simulink model "tmp_model_5"  (R2018b)
settings: Solver=VariableStepAuto  StartTime=0.0  StopTime=100  FixedStep=0.001  RelTol=1e-3
libraries: fl_lib x57, sdl_lib x18, nesl_utility x9
(part 1 of 3)
settings Model: Creator=Tanya  LastModifiedBy=Tanya
settings SolverCC: ZeroCrossAlgorithm=Adaptive
settings DebuggingCC: AlgebraicLoopMsg=none  MaskedZcDiagnostic=none  IgnoredZcDiagnostic=none

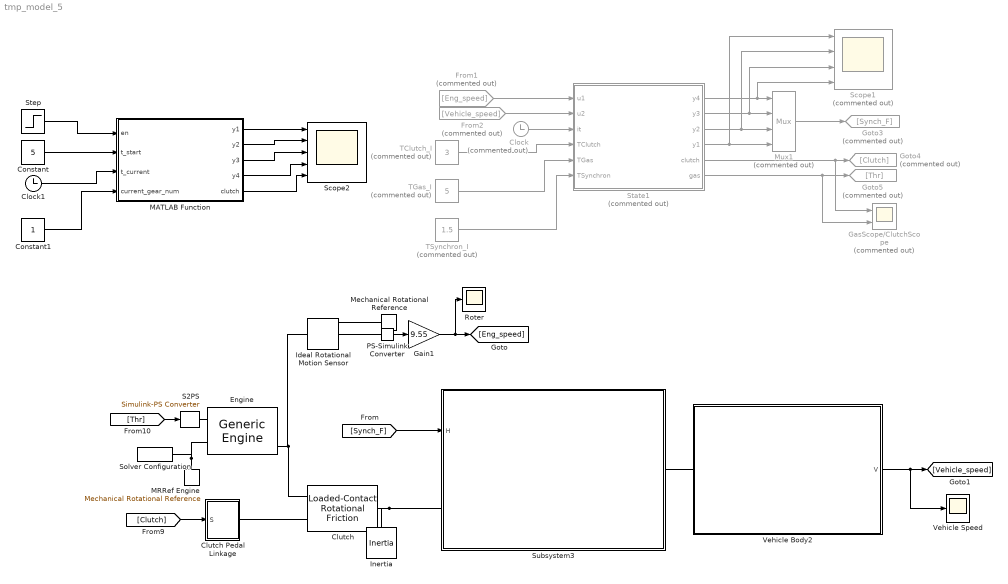
== system tmp_model_5 ==
  Clock : Clock  Commented=on
  Clock1 : Clock
  Clutch : sdl_lib/Brakes & Detents/Rotational/Loaded-Contact Rotational Friction  geometry_model=1  r_eff=300 mm  d_o=150 mm  d_i=100 mm  friction_model=1  mu_coulomb=0.46  mu_w_vector=[ 0 0.1 0.2 0.3 0.4 0.5 1 2 5 10 100 1000 ] rad/s  mu_coulomb_vector=[ 0.29 0.28 0.26 0.22 0.21 0.2 0.2 0.19 0.19 0.19 0.19 0.19 ]  mu_interp_method=1  mu_extrap_method=1  mu_static=0.5  w_tol=0.001 rad/s  force_min=10 N  mu_visc=0 N*m/(rad/s)  initial_state_locked=0  temperature_TLU=[280.0, 300.0, 320.0] K  mu_coulomb_temp_vector=[0.3, 0.28, 0.25]  mu_coulomb_matrix=[0.34, 0.32, 0.3; 0.3, 0.28, 0.25; 0.25, 0.2, 0.15]  mu_static_vector=[0.4, 0.38, 0.36]  thermal_mass=50 kJ/K  T_init=300 K
      settings: SourceProductName=Simscape Driveline  SourceProductBaseCode=LD
  Clutch Pedal Linkage : Subsystem  Tag=PublishSubsystem
      mask Display:
      | color('white')
      | plot(-40,-80);
      | plot(40,40);
      | color('black'),
      | patch([-45 -30 -20 -20 -45],[-90 -90 -75 -55 -90]+20)
      | patch([-30 -10  5 10 20 [20 10 6 -10 -30]-2],[-55 -50 20 25 35 fliplr([-55 -50 20 25 35])-5]);
  Constant : Constant  Value=5
  Constant1 : Constant
  Engine : sdl_lib/Engines/Generic Engine  model_parameterization=1  engine_type=1  P_max=100e3 W  w_P_max=6500 rpm  w_max=8500 rpm  w_min=200 rpm  w_tab=[ 500 1000 2e+3 3e+3 4e+3 5e+3 6e+3 7e+3 ] rpm  trq_tab=[ 380 380 380 380 350 280 200 80 ] N*m  pwr_tab=[ 2e+4 4e+4 7.8e+4 1.2e+5 1.45e+5 1.48e+5 1.25e+5 6e+4 ] W  interp_method=simscape.enum.interpolation.linear  model_inertia=1  inertia=0.16 kg*m^2  initial_velocity=800 rpm  model_time_constant=1  time_constant=0.2 s  T0=0  w_thr=20 rpm  idle_speed=1  idle_speed_reference=800 rpm  tau_controller=.6 s  idle_w_thr=1 rpm  redline=0  redline_speed=5000 rpm  tau_redline=1 s  redline_w_thr=1 rpm  fc_model=0  fc_per_rev=25 mg/rev  displaced_volume=400 cm^3  rev_per_cycle=2  fc_w_tab=[ 1000 2e+3 3e+3 4e+3 5e+3 6e+3 ] rpm  fc_trq_tab=[ 0 80 160 200 240 320 360 400 ] N*m  fc_tab=[ 0.5 0.9 1.4 1.6 1.9 2.7 3.4 4.4; 1 1.7 2.7 3.1 3.6 5 6 7.4; 1.4 2.7 4 4.8 5.6 7.5 8.5 10.5; 2 3.6 5.8 6.7 8 10.4 11.7 13.3; 2.5 4.8 7.9 9.4 10.8 14 16.2 18.6; 3.1 6 10.3 11.9 13.8 18.4 22 26.5 ] g/s  bmep_tab=[ 0 250 500 625 750 1000 1.15e+3 1.25e+3 ] kPa  bsfc_tab=[ 410 380 300 280 270 290 320 380; 410 370 290 270 260 270 285 320; 415 380 290 275 265 270 270 300; 420 390 310 290 285 280 280 285; 430 410 340 320 310 300 310 320; 450 430 370 340 330 330 350 380 ] g/hr/kW  fc_interp_method=simscape.enum.interpolation.linear
      settings: SourceProductName=Simscape Driveline  SourceProductBaseCode=LD
  From1 : From  Commented=on  GotoTag=Eng_speed
  From2 : From  Commented=on  GotoTag=Vehicle_speed
  Gain1 : Gain  Gain=9.55
  GasScope/ClutchScope : Scope  Commented=on  NumInputPorts=2
  Goto3 : Goto  Commented=on  GotoTag=Synch_F
  Goto4 : Goto  Commented=on  GotoTag=Clutch
  Goto5 : Goto  Commented=on  GotoTag=Thr
  Ideal Rotational Motion Sensor : fl_lib/Mechanical/Mechanical Sensors/Ideal Rotational Motion Sensor  offset=0 rad
  Inertia : fl_lib/Mechanical/Rotational Elements/Inertia  inertia=0.005 kg*m^2  w_specify=off  w_priority=High  w=0 rad/s  w_nominal_specify=off  w_nominal_unit=rad/s  w_nominal_value=1  t_specify=off  t_priority=High  t=0 N*m  t_nominal_specify=off  t_nominal_unit=N*m  t_nominal_value=1
  MATLAB Function : MATLAB Function  TreatAsAtomicUnit=on
  MRRef Engine : fl_lib/Mechanical/Rotational Elements/Mechanical Rotational Reference
  Mechanical Rotational Reference : fl_lib/Mechanical/Rotational Elements/Mechanical Rotational Reference
  Mux1 : Mux  Commented=on
  PS-Simulink Converter : nesl_utility/PS-Simulink Converter  PhysicalDomain=network_engine_domain  SubClassName=ps_output  LeftPortType=input  RightPortType=output  PseudoPeriodic=off  Frequencies=[]  Unit=rad/s  AffineConversion=off
  Roter : Scope
  S2PS : nesl_utility/Simulink-PS Converter  PhysicalDomain=network_engine_domain  SubClassName=ps_input  LeftPortType=input  RightPortType=output  PseudoPeriodic=off  Frequencies=[]  NoiseDistribution=none  NoiseParameters=[]  Unit=1  AffineConversion=off  FilteringAndDerivatives=zero  SimscapeFilterOrder=1  InputFilterTimeConstant=.001  UdotUserProvided=0
  Scope1 : Scope  Commented=on  NumInputPorts=4
  Scope2 : Scope  NumInputPorts=5
  Solver Configuration : nesl_utility/Solver Configuration  PhysicalDomain=network_engine_domain  SubClassName=solver  LeftPortType=input  RightPortType=generic  Tones=[]  Harmonics=[]  SimulateNoise=off  Profile=off  UseLocalSampling=off  EnableSwitchedLinearOptims=on  FrequencyDomain=off  UseCCode=off  RelTol=0.001  AbsTol=1e-06  MinStep=1e-09  ToWorkspace=off  RevertToSquareIcSolve=off  NumHomotopyIterations=100  PhasorMode=off  PhasorModeNumHarmonics=1  DoDC=off  ResidualTolerance=1e-9  UseLocalSolver=off  LocalSolverChoice=NE_BACKWARD_EULER_ADVANCER  LocalSolverSampleTime=.001  DoFixedCost=off  MaxNonlinIter=3  MaxModeIter=2  LinearAlgebra=auto  EquationFormulation=NE_TIME_EF  DelaysMemoryBudget=1024  AutomaticFiltering=on  FilteringTimeConstant=0.001  PartitionStorageMethod=AS_NEEDED  PartitionMemoryBudget=1024
  State1 : MATLAB Function  Commented=on  TreatAsAtomicUnit=on
  Step : Step  Time=5  SampleTime=0
  Subsystem3 : Subsystem
      mask Display: image('content_ponizhennaya_peredacha_nizhnyaya_stupen_delitelya2.png');
  TClutch_I : Constant  Commented=on  Value=3
  TGas_I : Constant  Commented=on  Value=5
  TSynchron_I : Constant  Commented=on  Value=1.5
  Vehicle Speed : Scope
  Vehicle Body2 : Subsystem  Tag=PublishSubsystem
      mask Display: image('gazel_avto.png');
  wires:
  [Thr] -> S2PS/1
  [Synch_F] -> Subsystem3/1(H)
  [Clutch] -> Clutch Pedal Linkage/1(S)
  PS-Simulink Converter/1 -> Gain1/1
  Clock/1 -> State1/3(it)
  Mux1/1 -> Goto3/1
  TClutch_I/1 -> State1/4(TClutch)
  TGas_I/1 -> State1/5(TGas)
  TSynchron_I/1 -> State1/6(TSynchron)
  Gain1/1 -> [Eng_speed], Roter/1
  State1/1(y4) -> Scope1/4, Mux1/1
  State1/2(y3) -> Scope1/3, Mux1/2
  State1/3(y2) -> Scope1/2, Mux1/3
  State1/4(y1) -> Scope1/1, Mux1/4
  State1/5(clutch) -> GasScope/ClutchScope/1, Goto4/1
  State1/6(gas) -> GasScope/ClutchScope/2, Goto5/1
  Vehicle Body2/1(V) -> [Vehicle_speed], Vehicle Speed/1
  From1/1 -> State1/1(u1)
  From2/1 -> State1/2(u2)
  Step/1 -> MATLAB Function/1(en)
  Constant/1 -> MATLAB Function/2(t_start)
  Clock1/1 -> MATLAB Function/3(t_current)
  Constant1/1 -> MATLAB Function/4(current_gear_num)
  MATLAB Function/1(y1) -> Scope2/1
  MATLAB Function/2(y2) -> Scope2/2
  MATLAB Function/3(y3) -> Scope2/3
  MATLAB Function/4(y4) -> Scope2/4
  MATLAB Function/5(clutch) -> Scope2/5
  connections:
  Clutch/RConn1 -- Inertia/LConn1 -- Subsystem3/LConn1
  MRRef Engine/LConn1 -- Solver Configuration/RConn1 -- Engine/LConn2
  Ideal Rotational Motion Sensor/LConn1 -- Clutch/LConn2 -- Engine/RConn3
  Clutch Pedal Linkage/RConn1 -- Clutch/LConn1
  Engine/LConn1 -- S2PS/RConn1
  Mechanical Rotational Reference/LConn1 -- Ideal Rotational Motion Sensor/RConn1
  PS-Simulink Converter/LConn1 -- Ideal Rotational Motion Sensor/RConn2
  Vehicle Body2/LConn1 -- Subsystem3/RConn1

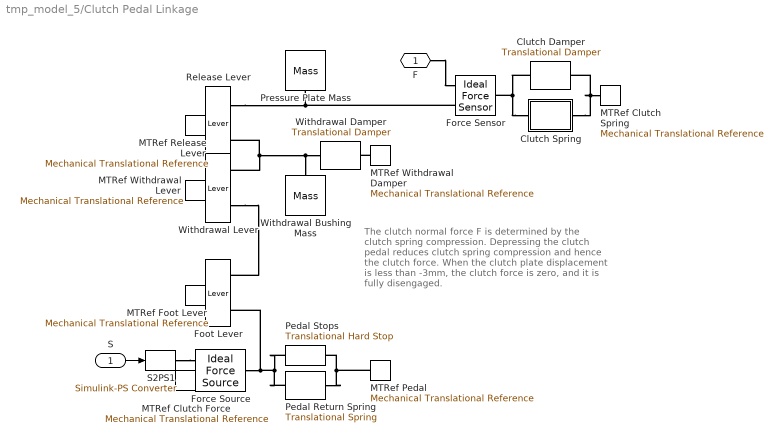
== system tmp_model_5/Clutch Pedal Linkage ==
  note: The clutch normal force F is determined by the
      | clutch spring compression. Depressing the
      | clutch pedal reduces clutch spring compression
      | and hence the clutch force. When the clutch plate
      | displacement is less than -3mm, the
      | clutch force is zero, and it is fully disengaged.
  S : Inport
  Clutch Damper : fl_lib/Mechanical/Translational Elements/Translational Damper  D=100 N/(m/s)  v_specify=off  v_priority=High  v=0 m/s  v_nominal_specify=off  v_nominal_unit=m/s  v_nominal_value=1  f_specify=off  f_priority=High  f=0 N  f_nominal_specify=off  f_nominal_unit=N  f_nominal_value=1
  Clutch Spring : Subsystem
  Foot Lever : fl_lib/Mechanical/Mechanisms/Lever  arm_AC=76 mm  arm_BC=148 mm  f_A_specify=off  f_A_priority=High  f_A=0 N  f_A_nominal_specify=off  f_A_nominal_unit=N  f_A_nominal_value=1  f_B_specify=off  f_B_priority=High  f_B=0 N  f_B_nominal_specify=off  f_B_nominal_unit=N  f_B_nominal_value=1  f_C_specify=off  f_C_priority=High  f_C=0 N  f_C_nominal_specify=off  f_C_nominal_unit=N  f_C_nominal_value=1
      settings: SourceProductName=Simscape  SourceProductBaseCode=SS
  Force Sensor : fl_lib/Mechanical/Mechanical Sensors/Ideal Force Sensor
  Force Source : fl_lib/Mechanical/Mechanical Sources/Ideal Force Source
  MTRef Clutch Force : fl_lib/Mechanical/Translational Elements/Mechanical Translational Reference
  MTRef Foot Lever : fl_lib/Mechanical/Translational Elements/Mechanical Translational Reference
  MTRef Release Lever : fl_lib/Mechanical/Translational Elements/Mechanical Translational Reference
  MTRef Withdrawal Damper : fl_lib/Mechanical/Translational Elements/Mechanical Translational Reference
  MTRef Withdrawal Lever : fl_lib/Mechanical/Translational Elements/Mechanical Translational Reference
  "MTRef Clutch Spring " : fl_lib/Mechanical/Translational Elements/Mechanical Translational Reference
  MTRef Pedal : fl_lib/Mechanical/Translational Elements/Mechanical Translational Reference
  Pedal Return Spring : fl_lib/Mechanical/Translational Elements/Translational Spring  spr_rate=120 N/m  v_specify=off  v_priority=High  v=0 m/s  v_nominal_specify=off  v_nominal_unit=m/s  v_nominal_value=1  f_specify=off  f_priority=High  f=0 N  f_nominal_specify=off  f_nominal_unit=N  f_nominal_value=1  x_specify=on  x_priority=High  x=1.5 cm  x_nominal_specify=off  x_nominal_unit=m  x_nominal_value=1
  Pedal Stops : fl_lib/Mechanical/Translational Elements/Translational Hard Stop  upper_bnd=168 mm  lower_bnd=0 mm  stiff_up=1e6 N/m  stiff_low=1e6 N/m  D_up=150 N/(m/s)  D_low=150 N/(m/s)  model=3  transition=0.1 mm  v_specify=off  v_priority=High  v=0 m/s  v_nominal_specify=off  v_nominal_unit=m/s  v_nominal_value=1  f_specify=off  f_priority=High  f=0 N  f_nominal_specify=off  f_nominal_unit=N  f_nominal_value=1  x_specify=off  x_priority=High  x=0 m  x_nominal_specify=off  x_nominal_unit=m  x_nominal_value=1
  Pressure Plate Mass : fl_lib/Mechanical/Translational Elements/Mass  mass=4.2 kg  v_specify=off  v_priority=High  v=0 m/s  v_nominal_specify=off  v_nominal_unit=m/s  v_nominal_value=1  f_specify=off  f_priority=High  f=0 N  f_nominal_specify=off  f_nominal_unit=N  f_nominal_value=1
  Release Lever : fl_lib/Mechanical/Mechanisms/Lever  arm_AC=7.2 mm  arm_BC=38 mm  f_A_specify=off  f_A_priority=High  f_A=0 N  f_A_nominal_specify=off  f_A_nominal_unit=N  f_A_nominal_value=1  f_B_specify=off  f_B_priority=High  f_B=0 N  f_B_nominal_specify=off  f_B_nominal_unit=N  f_B_nominal_value=1  f_C_specify=off  f_C_priority=High  f_C=0 N  f_C_nominal_specify=off  f_C_nominal_unit=N  f_C_nominal_value=1
      settings: SourceProductName=Simscape  SourceProductBaseCode=SS
  S2PS1 : nesl_utility/Simulink-PS Converter  PhysicalDomain=network_engine_domain  SubClassName=ps_input  LeftPortType=input  RightPortType=output  PseudoPeriodic=off  Frequencies=[]  NoiseDistribution=none  NoiseParameters=[]  Unit=1  AffineConversion=off  FilteringAndDerivatives=filter  SimscapeFilterOrder=1  InputFilterTimeConstant=.001  UdotUserProvided=0
  Withdrawal Bushing Mass : fl_lib/Mechanical/Translational Elements/Mass  mass=0.6 kg  v_specify=off  v_priority=High  v=0 m/s  v_nominal_specify=off  v_nominal_unit=m/s  v_nominal_value=1  f_specify=off  f_priority=High  f=0 N  f_nominal_specify=off  f_nominal_unit=N  f_nominal_value=1
  Withdrawal Lever : fl_lib/Mechanical/Mechanisms/Lever  arm_AC=42 mm  arm_BC=128 mm  f_A_specify=off  f_A_priority=High  f_A=0 N  f_A_nominal_specify=off  f_A_nominal_unit=N  f_A_nominal_value=1  f_B_specify=off  f_B_priority=High  f_B=0 N  f_B_nominal_specify=off  f_B_nominal_unit=N  f_B_nominal_value=1  f_C_specify=off  f_C_priority=High  f_C=0 N  f_C_nominal_specify=off  f_C_nominal_unit=N  f_C_nominal_value=1
      settings: SourceProductName=Simscape  SourceProductBaseCode=SS
  Withdrawal Damper : fl_lib/Mechanical/Translational Elements/Translational Damper  D=100 N/(m/s)  v_specify=off  v_priority=High  v=0 m/s  v_nominal_specify=off  v_nominal_unit=m/s  v_nominal_value=1  f_specify=off  f_priority=High  f=0 N  f_nominal_specify=off  f_nominal_unit=N  f_nominal_value=1
  F : PMIOPort  Side=Right
  wires:
  S/1 -> S2PS1/1
  connections:
  MTRef Foot Lever/LConn1 -- Foot Lever/RConn1
  MTRef Pedal/LConn1 -- Pedal Return Spring/RConn1 -- Pedal Stops/RConn1
  MTRef Withdrawal Damper/LConn1 -- Withdrawal Damper/RConn1
  MTRef Release Lever/LConn1 -- Release Lever/RConn1
  Withdrawal Lever/LConn2 -- Foot Lever/LConn1
  MTRef Withdrawal Lever/LConn1 -- Withdrawal Lever/RConn1
  Withdrawal Lever/LConn1 -- Release Lever/LConn2 -- Withdrawal Bushing Mass/LConn1 -- Withdrawal Damper/LConn1
  Release Lever/LConn1 -- Force Sensor/RConn1 -- Pressure Plate Mass/LConn1
  Pedal Stops/LConn1 -- Pedal Return Spring/LConn1 -- Force Source/LConn1 -- Foot Lever/LConn2
  "MTRef Clutch Spring "/LConn1 -- Clutch Spring/RConn1 -- Clutch Damper/RConn1
  Clutch Spring/LConn1 -- Clutch Damper/LConn1 -- Force Sensor/LConn1
  F/RConn1 -- Force Sensor/RConn2
  MTRef Clutch Force/LConn1 -- Force Source/RConn2
  S2PS1/RConn1 -- Force Source/RConn1
